simulink model "erc_vision_node"  (R2026a)
settings: Solver=FixedStepDiscrete  StopTime=inf  FixedStep=1/15  EnableMultiTasking=on
undefined symbols (not defined in the file or in its folder): x, y, z
libraries: ros2lib x2, raspberrypiAVlib x1
settings Model: Creator=Marko  LastModifiedBy=yagodanr
settings SolverCC: PositivePriorityOrder=on
settings HardwareCC: ProdBitPerLong=64.0  ProdLargestAtomicInteger=LongLong  ProdLargestAtomicFloat=Double  ProdHWDeviceType=ARM Compatible->ARM Cortex-A (64-bit)
settings SFSimCC: SimTargetLang=C++
settings RTWCC: SystemTargetFile=ert.tlc  HardwareBoard=Robot Operating System 2 (ROS 2)  TLCOptions="-aInlineSetEventsForThisBaseRateFcn=TLC_FALSE -aSuppressMultiTaskScheduler=TLC_FALSE  -aRateBasedStepFcn=0"  Toolchain=Colcon Tools  TargetLang=C++  Description=Embedded Coder
settings ERTTargetCC: ExtModeTransport=2.0  ExtModeAutomaticAllocSize=off  RootIOFormat=Structure reference  CodeInterfacePackaging=C++ class  SupportVariableSizeSignals=on

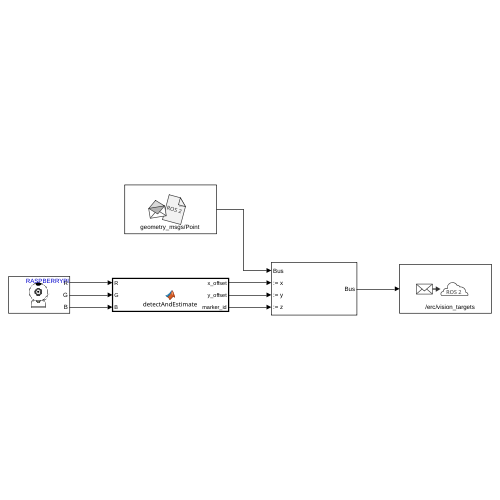
[thumbnail: Simulink's stored preview of the top-level diagram]
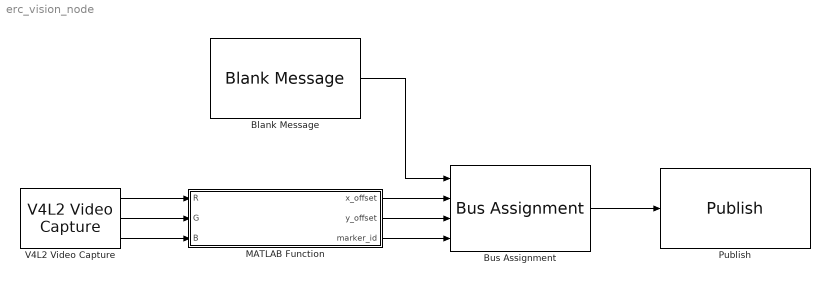
== system erc_vision_node ==
  Blank Message : ros2lib/Blank Message  messageClass=Message  entityType=geometry_msgs/Point  messageType=geometry_msgs/Point  SampleTime=inf
  Bus Assignment : BusAssignment  AssignedSignals=x,y,z
  MATLAB Function : MATLAB Function  TreatAsAtomicUnit=on
  Publish : ros2lib/Publish  topicSource=Specify your own  topic=/erc/vision_targets  messageType=geometry_msgs/Point  QOSHistory=Keep last  QOSDepth=10  QOSReliability=Reliable  QOSDurability=Volatile  QOSDeadline=Inf  QOSLifespan=Inf  QOSLiveliness=Automatic  QOSLeaseDuration=Inf  QOSAvoidROSNamespaceConventions=off
  V4L2 Video Capture : raspberrypiAVlib/V4L2 Video Capture  DeviceName=/dev/video10  Resolution=640x480  CustomResolution=[ 320, 240 ]  PixelFormat=RGB  SampleTime=1/15  pixelOrder=planar  simOutput=Colorbars  imSizeSelection=320x240  imSize=[640, 480]  roi=[0, 0, 640, 480]  m_devName='/dev/video0'  blockPlatform=LINUX  HorizontalFlip=off  VerticalFlip=off  Brightness=0.5  Saturation=0.5  Contrast=0.5  Sharpness=0.5  CameraPan=0  CameraTilt=0  CameraZoom=0.5  EnableManualFocus=off  ManualFocus=0.5
  wires:
  V4L2 Video Capture/1 -> MATLAB Function/1(R)
  V4L2 Video Capture/2 -> MATLAB Function/2(G)
  V4L2 Video Capture/3 -> MATLAB Function/3(B)
  MATLAB Function/1(x_offset) -> Bus Assignment/2
  MATLAB Function/2(y_offset) -> Bus Assignment/3
  MATLAB Function/3(marker_id) -> Bus Assignment/4
  Bus Assignment/1 -> Publish/1
  Blank Message/1 -> Bus Assignment/1

== matlab function erc_vision_node/MATLAB Function ==
  data: R input; x_offset output; y_offset output; marker_id output; G input; B input
function [x_offset, y_offset, marker_id] = detectAndEstimate(R, G, B)
%#codegen

% ── Combine R, G, B planes into RGB image ──

if size(R,1) == 640 && size(R,2) == 480
    R_plane = R';
    G_plane = G';
    B_plane = B';
else
    R_plane = R;
    G_plane = G;
    B_plane = B;
end

frame = cat(3, R_plane, G_plane, B_plane);

% ── Camera intrinsics ──

focalLength    = [530.0, 530.0];
principalPoint = [320.0, 240.0];

% Keep this fixed for code generation.
imageSize = [480, 640];

intrinsics = cameraIntrinsics( ...
    focalLength, ...
    principalPoint, ...
    imageSize);

% ── Marker parameters ──

markerSizeMeters = 0.15;

% ── Default output ──

x_offset  = 0.0;
y_offset  = 0.0;
marker_id = 0.0;

% ── Detect + estimate pose in ONE operation ──

[ids, ~, poses] = readArucoMarker( ...
    frame, ...
    "DICT_ARUCO_ORIGINAL", ...
    intrinsics, ...
    markerSizeMeters);

% No markers
if isempty(ids)
    return;
end

% ── Priority: 102 > 101 ──

targetIdx = 0;

for i = 1:numel(ids)
    if ids(i) == 102
        targetIdx = i;
        break;
    end
end

if targetIdx == 0
    for i = 1:numel(ids)
        if ids(i) == 101
            targetIdx = i;
            break;
        end
    end
end

% Ignore markers other than 101/102
if targetIdx == 0
    return;
end

% ── Extract marker translation ──

tvec = poses(targetIdx).Translation;

x_offset  = tvec(1);
y_offset  = tvec(2);
marker_id = double(ids(targetIdx));

end
